simulink model "Ejer4_PrestamoBalance"  (R2023b)
settings: Solver=FixedStepDiscrete  StartTime=0  StopTime=100  FixedStep=1  RelTol=1e-3
undefined symbols (not defined in the file): b0, DiscIntNeverNeededParam, it, p
settings Model: Creator=alfre  LastModifiedBy=alfre

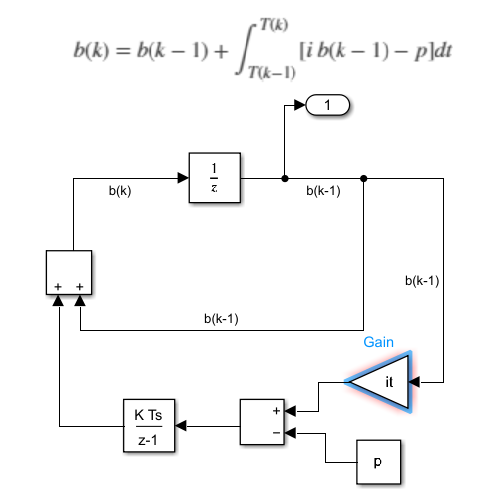
[thumbnail: Simulink's stored preview of the top-level diagram]
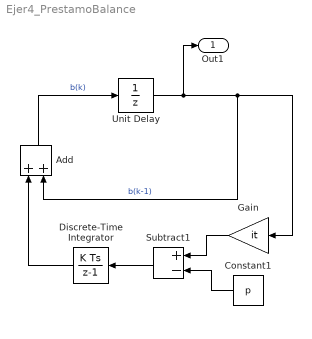
== system Ejer4_PrestamoBalance ==
  Add : Sum
  Constant1 : Constant  Value=p
  Discrete-Time Integrator : DiscreteIntegrator  gainval=1  SampleTime=-1  ICPrevOutput=DiscIntNeverNeededParam  ICPrevScaledInput=DiscIntNeverNeededParam
  Gain : Gain  Gain=it
  Subtract1 : Sum  Inputs=+-
  Unit Delay : UnitDelay  InitialCondition=b0  SampleTime=-1  HasFrameUpgradeWarning=on
  Out1 : Outport
  wires:
  Unit Delay/1 -> Out1/1, Add/2, Gain/1  "b(k-1)"
  Gain/1 -> Subtract1/1
  Constant1/1 -> Subtract1/2
  Subtract1/1 -> Discrete-Time Integrator/1
  Discrete-Time Integrator/1 -> Add/1
  Add/1 -> Unit Delay/1  "b(k)"
